simulink model "Reator_inrunsh"  (R2021a)
settings: Solver=ode23tb  StartTime=0.0  StopTime=3  RelTol=1e-6  AbsTol=1e-6
InitFcn:
  | R0 = 1e-6
  | R1 = R0
  | R2 = R0
  | R3 = R0
  | R4 = R0
  | R5 = R0
  | R6 = R0
  | 
  | L0 = 222.79e-6
  | L1 = L0
  | L2 = L0
  | L3 = L0
  | L4 = L0
  | L5 = L0
  | L6 = L0
  | 
  | C0 = 60.17e-6
  | C1 = C0
  | C2 = C0
  | C3 = C0
  | C4 = C0
  | C5 = C0
  | C6 = C0
libraries: spsSeriesRLCBranchLib x8, spsACVoltageSourceLib x1, spsBreakerLib x1, spsMultimeterLib x1, spsRMSLib x1, spspowerguiLib x1
settings Model: Creator=angel  LastModifiedBy=angel
settings DebuggingCC: UnconnectedInputMsg=none  UnconnectedOutputMsg=none  UnconnectedLineMsg=none

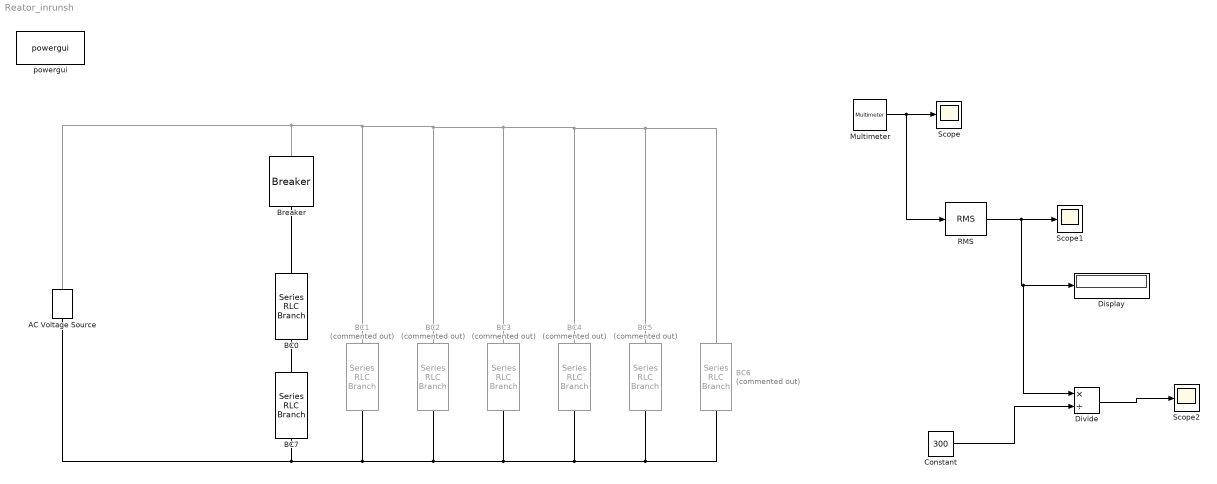
== system Reator_inrunsh ==
  AC Voltage Source : spsACVoltageSourceLib/AC Voltage Source  Amplitude=23.1e3 *sqrt(2/3)  Phase=0  Frequency=60  SampleTime=0  Measurements=None  BusType=swing  Pref=10e3  Qref=0  Qmin=-inf  Qmax=+inf
  BC0 : spsSeriesRLCBranchLib/Series RLC Branch  LConnTagsString=__new0  RConnTagsString=__new0  BranchType=RL  Resistance=R0  Inductance=L0*10  SetiL0=on  InitialCurrent=0  Capacitance=C0  Setx0=off  InitialVoltage=0  Measurements=None
  BC1 : spsSeriesRLCBranchLib/Series RLC Branch  Commented=on  LConnTagsString=__new0  RConnTagsString=__new0  BranchType=RLC  Resistance=R1  Inductance=L1  SetiL0=off  InitialCurrent=0  Capacitance=C1  Setx0=off  InitialVoltage=0  Measurements=None
  BC2 : spsSeriesRLCBranchLib/Series RLC Branch  Commented=on  LConnTagsString=__new0  RConnTagsString=__new0  BranchType=RLC  Resistance=R2  Inductance=L2  SetiL0=off  InitialCurrent=0  Capacitance=C2  Setx0=off  InitialVoltage=0  Measurements=None
  BC3 : spsSeriesRLCBranchLib/Series RLC Branch  Commented=on  LConnTagsString=__new0  RConnTagsString=__new0  BranchType=RLC  Resistance=R3  Inductance=L3  SetiL0=off  InitialCurrent=0  Capacitance=C3  Setx0=off  InitialVoltage=0  Measurements=None
  BC4 : spsSeriesRLCBranchLib/Series RLC Branch  Commented=on  LConnTagsString=__new0  RConnTagsString=__new0  BranchType=RLC  Resistance=R4  Inductance=L4  SetiL0=off  InitialCurrent=0  Capacitance=C4  Setx0=off  InitialVoltage=0  Measurements=None
  BC5 : spsSeriesRLCBranchLib/Series RLC Branch  Commented=on  LConnTagsString=__new0  RConnTagsString=__new0  BranchType=RLC  Resistance=R5  Inductance=L5  SetiL0=off  InitialCurrent=0  Capacitance=C5  Setx0=off  InitialVoltage=0  Measurements=None
  BC6 : spsSeriesRLCBranchLib/Series RLC Branch  Commented=on  LConnTagsString=__new0  RConnTagsString=__new0  BranchType=RLC  Resistance=R6  Inductance=L6  SetiL0=off  InitialCurrent=0  Capacitance=C6  Setx0=off  InitialVoltage=0  Measurements=None
  BC7 : spsSeriesRLCBranchLib/Series RLC Branch  LConnTagsString=__new0  RConnTagsString=__new0  BranchType=C  Resistance=R0  Inductance=L0  SetiL0=off  InitialCurrent=0  Capacitance=C0  Setx0=on  InitialVoltage=0  Measurements=Branch voltage and current
  Breaker : spsBreakerLib/Breaker  InitialState=0  SwitchingTimes=[1.25/60]  External=off  BreakerResistance=0.01  SnubberResistance=1e6  SnubberCapacitance=inf  Measurements=None  MoreParameters=on  NoBreakLoop=off
      settings: SourceProductBaseCode=PS
  Constant : Constant  Value=300
  Display : Display
  Divide : Product  Inputs=*/
  Multimeter : spsMultimeterLib/Multimeter  PhasorSimulation=off  OutputType=Complex  sel=[2 1]  L=2  Gain=[1 1]  yselected={'Ib: BC7','Ub: BC7'};  PSBOutputType=1  PSBequivalent=0  AxesSetting=[0,0.1,-100,100]  Display=1  SavedBlockNames=-11
  RMS : spsRMSLib/RMS  TrueRMS=on  Freq=60  RMSInit=120  Ts=0
  Scope : Scope
  Scope1 : Scope
  Scope2 : Scope
  powergui : spspowerguiLib/powergui  Priority=1  SimulationMode=Continuous  SampleTime=50e-6  frequency=60  Iterations=50  frequencyindice=60  Pbase=100e6  ErrMax=1e-4  UnitsV=kV  UnitsW=MW  buscounter=0  FunctionMessages=off  echomessages=off  EnableUseOfTLC=off  CurrentSourceSwitches=off  DisableSnubberDevices=off  DisableRonSwitches=off  DisableVfSwitches=off  DisplayEquations=off  AutomaticDiscreteSolvers=off  SolverType=Tustin/Backward Euler (TBE)  Interpol=off  ExternalGateDelay=off  methode=off  Ts=100  x0status=blocks  SPID=on  SwTol=0  HookPort=off  NonlinearTolerance=1e-4  nMaxIteration=100  ContinueOnMaxIteration=off  RestoreLinks=warning  ResistiveCurrentMeasurement=off  Frange=[0:2:500]  Ylog=off  Xlog=on  ShowGrid=off  save=off  variable=ZData  structure=0  ZoomFFT=off  StartTime=0.0  cycles=1  DisplayStyle=1  fundamental=60  FreqAxis=off  MaxFrequency=1000  frequencyindicesteady=1  RmsSteady=1  display=off
  wires:
  Multimeter/1 -> RMS/1, Scope/1
  RMS/1 -> Divide/1, Display/1, Scope1/1
  Constant/1 -> Divide/2
  Divide/1 -> Scope2/1
  connections:
  BC1/LConn1 -- BC6/LConn1 -- BC5/LConn1 -- BC4/LConn1 -- BC3/LConn1 -- BC2/LConn1 -- AC Voltage Source/RConn1 -- Breaker/LConn1
  AC Voltage Source/LConn1 -- BC7/RConn1 -- BC1/RConn1 -- BC2/RConn1 -- BC3/RConn1 -- BC4/RConn1 -- BC5/RConn1 -- BC6/RConn1
  BC0/LConn1 -- Breaker/RConn1
  BC0/RConn1 -- BC7/LConn1
